simulink model "building_EXAMPLE_v1"  (R2016b)
settings: Solver=ode23tb  StartTime=-building.preruntime+8760*3600  StopTime=building.runtime+8760*3600  MaxStep=600  EnableMultiTasking=on
StartFcn:
  | tic
StopFcn:
  | toc
values from neighbouring files (symbols this model uses):
  building = create_building_automatic(building, modify, import_mode, name_XML, name_EXCEL, name_PHPP, NUMBEROFZONES)    [work_EXAMPLE_v1.m]
undefined symbols (not defined in the file or in its folder): A, B, C, cp, Dd, Dreifach, FluidMix, get_building, ID, MassFlow, p, Pressure, Qdot_C, Qdot_C_energy, Qdot_H, Qdot_H_energy, Qdot_I_electricity, Qdot_I_electricity_energy, Qdot_I_light, Qdot_I_light_energy, Qdot_I_person, Qdot_I_person_energy, Qdot_S, Qdot_S_energy, Qdot_T_ground, Qdot_T_ground_energy, Qdot_T_neighbour, Qdot_T_neighbour_energy, Qdot_T_opaque, Qdot_T_opaque_energy, Qdot_T_window, Qdot_T_window_energy, Qdot_V_infiltration, Qdot_V_infiltration_energy, Qdot_V_mech, Qdot_V_mech_energy, Qdot_V_window, Qdot_V_window_energy, rho, Tc, Temperature, Tr, Ts, Wärmeschutzglas, x_CO2, x_H2O, x_VOC
libraries: carnotUIBK x1931, carnot x83, simulink_extras x22, simulink x12
(part 11 of 35)

== system building_EXAMPLE_v1/HVAC PKOM4/electrical heater 3 ==
  temperature room : Inport
  " " : Constant  Value=0
  "   " : Constant  Value=zeros(1,15)
  Bus Selector5 : BusSelector  OutputSignals=Ts
  Constant 3 : Constant  Value=theta_r_t  VectorParams1D=off
  Constant 9 : Constant  Value=theta_r_t_low  VectorParams1D=off
  Mux1 : Mux  Inputs=[1 1 15 1 1]
  PID_1 : simulink/Continuous/PID Controller  Controller=PI  TimeDomain=Continuous-time  SampleTime=-1  IntegratorMethod=Forward Euler  FilterMethod=Forward Euler  Form=Ideal  UseFilter=on  ControllerParametersSource=internal  P=Kp  I=(1/(Tn*60))  D=0  N=100  InitialConditionSource=internal  InitialConditionForIntegrator=0  InitialConditionForFilter=0  ExternalReset=none  LimitOutput=on  UpperSaturationLimit=1  LowerSaturationLimit=0  LinearizeAsGain=off  AntiWindupMode=clamping  Kb=1  TrackingMode=off  Kt=1  PParamMin=[]  PParamMax=[]  IParamMin=[]  IParamMax=[]  DParamMin=[]  DParamMax=[]  NParamMin=[]  NParamMax=[]  KbParamMin=[]  KbParamMax=[]  KtParamMin=[]  KtParamMax=[]  POutMin=[]  POutMax=[]  IOutMin=[]  IOutMax=[]  DOutMin=[]  DOutMax=[]  NOutMin=[]  NOutMax=[]  KbOutMin=[]  KbOutMax=[]  KtOutMin=[]  KtOutMax=[]  IntegratorOutMin=[]  IntegratorOutMax=[]  FilterOutMin=[]  FilterOutMax=[]  SumOutMin=[]  SumOutMax=[]  SumI1OutMin=[]  SumI1OutMax=[]  SumI2OutMin=[]  SumI2OutMax=[]  SumI3OutMin=[]  SumI3OutMax=[]  SumDOutMin=[]  SumDOutMax=[]  SaturationOutMin=[]  SaturationOutMax=[]  IntegratorContinuousStateAttributes=''  IntegratorStateMustResolveToSignalObject=off  IntegratorRTWStateStorageClass=Auto  FilterContinuousStateAttributes=''  FilterStateMustResolveToSignalObject=off  FilterRTWStateStorageClass=Auto  DifferentiatorICPrevScaledInput=0  DifferentiatorOutMin=[]  DifferentiatorOutMax=[]
  Sum13 : Sum  Inputs=|+-
  Switch : Switch  Criteria=u2 ~= 0
  Transfer Fcn (with initial states) : Subsystem  mask(Transfer Function with Initial States){N=[1], D=[timeconstant_heater  1], X0=0}
      mask prompts: N "Numerator:"; D "Denominator:"; X0 "Initial conditions:"
      mask help: Vector expressions for numerator, and denominator. Coefficients are in descending powers of s.
      mask init:
      | [A,B,C,Dd]=tf2ss(N,D);if (isempty(X0));[m,n]=size(A);X0=zeros(1,m); end;
      mask Help: Specify the initial states for the transfer function.  The state ordering is determined by the m-file tf2ss.  There is no unique mapping of the states in a transfer function to states in a state-space representation.  However, tf2ss will consistently use the same mapping for a given transfer function.
      mask Display: dpoly(N,D,'s')
  Transfer Fcn (with initial states)6 : Subsystem  mask(Transfer Function with Initial States){N=[1], D=[60  1], X0=0}
      mask prompts: N "Numerator:"; D "Denominator:"; X0 "Initial conditions:"
      mask help: Vector expressions for numerator, and denominator. Coefficients are in descending powers of s.
      mask init:
      | [A,B,C,Dd]=tf2ss(N,D);if (isempty(X0));[m,n]=size(A);X0=zeros(1,m); end;
      mask Help: Specify the initial states for the transfer function.  The state ordering is determined by the m-file tf2ss.  There is no unique mapping of the states in a transfer function to states in a state-space representation.  However, tf2ss will consistently use the same mapping for a given transfer function.
      mask Display: dpoly(N,D,'s')
  conv : Gain  Gain=1-part_rad  SaturateOnIntegerOverflow=on  OutDataTypeStr=Inherit: Same as input  ParamDataTypeStr=Inherit: Same as input
  heater : Product
  maximal power : Constant  Value=max_power
  rad : Gain  Gain=part_rad  SaturateOnIntegerOverflow=on  OutDataTypeStr=Inherit: Same as input  ParamDataTypeStr=Inherit: Same as input
  time profile : carnot/Load/General/Repeating_Profile  period=sum(control_time_duration)  rep_seq_t=control_time_values  rep_seq_d=control_time_duration  rep_seq_y=control_time_output
  "[S]" : Outport
  Pel : Outport  Port=2
  wires:
  time profile/1 -> Switch/2
  Switch/1 -> Sum13/1
  Constant 9/1 -> Switch/3
  Constant 3/1 -> Switch/1
  Transfer Fcn (with initial states)/1(Out1) -> Mux1/4, rad/1, conv/1
  Bus Selector5/1 -> Sum13/2  "<Ts>"
  Sum13/1 -> Transfer Fcn (with initial states)6/1(In1)
  heater/1 -> Transfer Fcn (with initial states)/1(In1), Pel/1
  "   "/1 -> Mux1/3
  rad/1 -> Mux1/2
  temperature room/1 -> Bus Selector5/1
  maximal power/1 -> heater/2
  conv/1 -> Mux1/1
  Mux1/1 -> "[S]"/1
  " "/1 -> Mux1/5
  PID_1/1 -> heater/1
  Transfer Fcn (with initial states)6/1(Out1) -> PID_1/1

== system building_EXAMPLE_v1/HVAC PKOM4/electrical heater 4 CONVECTOR ==
  temperature room : Inport
  " " : Constant  Value=0
  "   " : Constant  Value=zeros(1,15)
  Bus Selector5 : BusSelector  OutputSignals=Ts
  Constant 3 : Constant  Value=theta_r_t  VectorParams1D=off
  Constant 9 : Constant  Value=theta_r_t_low  VectorParams1D=off
  Mux1 : Mux  Inputs=[1 1 15 1 1]
  PID_1 : simulink/Continuous/PID Controller  Controller=PI  TimeDomain=Continuous-time  SampleTime=-1  IntegratorMethod=Forward Euler  FilterMethod=Forward Euler  Form=Ideal  UseFilter=on  ControllerParametersSource=internal  P=Kp  I=(1/(Tn*60))  D=0  N=100  InitialConditionSource=internal  InitialConditionForIntegrator=0  InitialConditionForFilter=0  ExternalReset=none  LimitOutput=on  UpperSaturationLimit=1  LowerSaturationLimit=0  LinearizeAsGain=off  AntiWindupMode=clamping  Kb=1  TrackingMode=off  Kt=1  PParamMin=[]  PParamMax=[]  IParamMin=[]  IParamMax=[]  DParamMin=[]  DParamMax=[]  NParamMin=[]  NParamMax=[]  KbParamMin=[]  KbParamMax=[]  KtParamMin=[]  KtParamMax=[]  POutMin=[]  POutMax=[]  IOutMin=[]  IOutMax=[]  DOutMin=[]  DOutMax=[]  NOutMin=[]  NOutMax=[]  KbOutMin=[]  KbOutMax=[]  KtOutMin=[]  KtOutMax=[]  IntegratorOutMin=[]  IntegratorOutMax=[]  FilterOutMin=[]  FilterOutMax=[]  SumOutMin=[]  SumOutMax=[]  SumI1OutMin=[]  SumI1OutMax=[]  SumI2OutMin=[]  SumI2OutMax=[]  SumI3OutMin=[]  SumI3OutMax=[]  SumDOutMin=[]  SumDOutMax=[]  SaturationOutMin=[]  SaturationOutMax=[]  IntegratorContinuousStateAttributes=''  IntegratorStateMustResolveToSignalObject=off  IntegratorRTWStateStorageClass=Auto  FilterContinuousStateAttributes=''  FilterStateMustResolveToSignalObject=off  FilterRTWStateStorageClass=Auto  DifferentiatorICPrevScaledInput=0  DifferentiatorOutMin=[]  DifferentiatorOutMax=[]
  Sum13 : Sum  Inputs=|+-
  Switch : Switch  Criteria=u2 ~= 0
  Transfer Fcn (with initial states) : Subsystem  mask(Transfer Function with Initial States){N=[1], D=[timeconstant_heater  1], X0=0}
      mask prompts: N "Numerator:"; D "Denominator:"; X0 "Initial conditions:"
      mask help: Vector expressions for numerator, and denominator. Coefficients are in descending powers of s.
      mask init:
      | [A,B,C,Dd]=tf2ss(N,D);if (isempty(X0));[m,n]=size(A);X0=zeros(1,m); end;
      mask Help: Specify the initial states for the transfer function.  The state ordering is determined by the m-file tf2ss.  There is no unique mapping of the states in a transfer function to states in a state-space representation.  However, tf2ss will consistently use the same mapping for a given transfer function.
      mask Display: dpoly(N,D,'s')
  Transfer Fcn (with initial states)6 : Subsystem  mask(Transfer Function with Initial States){N=[1], D=[60  1], X0=0}
      mask prompts: N "Numerator:"; D "Denominator:"; X0 "Initial conditions:"
      mask help: Vector expressions for numerator, and denominator. Coefficients are in descending powers of s.
      mask init:
      | [A,B,C,Dd]=tf2ss(N,D);if (isempty(X0));[m,n]=size(A);X0=zeros(1,m); end;
      mask Help: Specify the initial states for the transfer function.  The state ordering is determined by the m-file tf2ss.  There is no unique mapping of the states in a transfer function to states in a state-space representation.  However, tf2ss will consistently use the same mapping for a given transfer function.
      mask Display: dpoly(N,D,'s')
  conv : Gain  Gain=1-part_rad  SaturateOnIntegerOverflow=on  OutDataTypeStr=Inherit: Same as input  ParamDataTypeStr=Inherit: Same as input
  heater : Product
  maximal power : Constant  Value=max_power
  rad : Gain  Gain=part_rad  SaturateOnIntegerOverflow=on  OutDataTypeStr=Inherit: Same as input  ParamDataTypeStr=Inherit: Same as input
  time profile : carnot/Load/General/Repeating_Profile  period=sum(control_time_duration)  rep_seq_t=control_time_values  rep_seq_d=control_time_duration  rep_seq_y=control_time_output
  "[S]" : Outport
  Pel : Outport  Port=2
  wires:
  Transfer Fcn (with initial states)6/1(Out1) -> PID_1/1
  PID_1/1 -> heater/1
  " "/1 -> Mux1/5
  Mux1/1 -> "[S]"/1
  conv/1 -> Mux1/1
  maximal power/1 -> heater/2
  temperature room/1 -> Bus Selector5/1
  rad/1 -> Mux1/2
  "   "/1 -> Mux1/3
  heater/1 -> Pel/1, Transfer Fcn (with initial states)/1(In1)
  Sum13/1 -> Transfer Fcn (with initial states)6/1(In1)
  Bus Selector5/1 -> Sum13/2  "<Ts>"
  Transfer Fcn (with initial states)/1(Out1) -> conv/1, rad/1, Mux1/4
  Constant 3/1 -> Switch/1
  Constant 9/1 -> Switch/3
  Switch/1 -> Sum13/1
  time profile/1 -> Switch/2

== system building_EXAMPLE_v1/HVAC PKOM4/electrical heater 5 ==
  temperature room : Inport
  " " : Constant  Value=0
  "   " : Constant  Value=zeros(1,15)
  Bus Selector5 : BusSelector  OutputSignals=Ts
  Constant 3 : Constant  Value=theta_r_t  VectorParams1D=off
  Constant 9 : Constant  Value=theta_r_t_low  VectorParams1D=off
  Mux1 : Mux  Inputs=[1 1 15 1 1]
  PID_1 : simulink/Continuous/PID Controller  Controller=PI  TimeDomain=Continuous-time  SampleTime=-1  IntegratorMethod=Forward Euler  FilterMethod=Forward Euler  Form=Ideal  UseFilter=on  ControllerParametersSource=internal  P=Kp  I=(1/(Tn*60))  D=0  N=100  InitialConditionSource=internal  InitialConditionForIntegrator=0  InitialConditionForFilter=0  ExternalReset=none  LimitOutput=on  UpperSaturationLimit=1  LowerSaturationLimit=0  LinearizeAsGain=off  AntiWindupMode=clamping  Kb=1  TrackingMode=off  Kt=1  PParamMin=[]  PParamMax=[]  IParamMin=[]  IParamMax=[]  DParamMin=[]  DParamMax=[]  NParamMin=[]  NParamMax=[]  KbParamMin=[]  KbParamMax=[]  KtParamMin=[]  KtParamMax=[]  POutMin=[]  POutMax=[]  IOutMin=[]  IOutMax=[]  DOutMin=[]  DOutMax=[]  NOutMin=[]  NOutMax=[]  KbOutMin=[]  KbOutMax=[]  KtOutMin=[]  KtOutMax=[]  IntegratorOutMin=[]  IntegratorOutMax=[]  FilterOutMin=[]  FilterOutMax=[]  SumOutMin=[]  SumOutMax=[]  SumI1OutMin=[]  SumI1OutMax=[]  SumI2OutMin=[]  SumI2OutMax=[]  SumI3OutMin=[]  SumI3OutMax=[]  SumDOutMin=[]  SumDOutMax=[]  SaturationOutMin=[]  SaturationOutMax=[]  IntegratorContinuousStateAttributes=''  IntegratorStateMustResolveToSignalObject=off  IntegratorRTWStateStorageClass=Auto  FilterContinuousStateAttributes=''  FilterStateMustResolveToSignalObject=off  FilterRTWStateStorageClass=Auto  DifferentiatorICPrevScaledInput=0  DifferentiatorOutMin=[]  DifferentiatorOutMax=[]
  Sum13 : Sum  Inputs=|+-
  Switch : Switch  Criteria=u2 ~= 0
  Transfer Fcn (with initial states) : Subsystem  mask(Transfer Function with Initial States){N=[1], D=[timeconstant_heater  1], X0=0}
      mask prompts: N "Numerator:"; D "Denominator:"; X0 "Initial conditions:"
      mask help: Vector expressions for numerator, and denominator. Coefficients are in descending powers of s.
      mask init:
      | [A,B,C,Dd]=tf2ss(N,D);if (isempty(X0));[m,n]=size(A);X0=zeros(1,m); end;
      mask Help: Specify the initial states for the transfer function.  The state ordering is determined by the m-file tf2ss.  There is no unique mapping of the states in a transfer function to states in a state-space representation.  However, tf2ss will consistently use the same mapping for a given transfer function.
      mask Display: dpoly(N,D,'s')
  Transfer Fcn (with initial states)6 : Subsystem  mask(Transfer Function with Initial States){N=[1], D=[60  1], X0=0}
      mask prompts: N "Numerator:"; D "Denominator:"; X0 "Initial conditions:"
      mask help: Vector expressions for numerator, and denominator. Coefficients are in descending powers of s.
      mask init:
      | [A,B,C,Dd]=tf2ss(N,D);if (isempty(X0));[m,n]=size(A);X0=zeros(1,m); end;
      mask Help: Specify the initial states for the transfer function.  The state ordering is determined by the m-file tf2ss.  There is no unique mapping of the states in a transfer function to states in a state-space representation.  However, tf2ss will consistently use the same mapping for a given transfer function.
      mask Display: dpoly(N,D,'s')
  conv : Gain  Gain=1-part_rad  SaturateOnIntegerOverflow=on  OutDataTypeStr=Inherit: Same as input  ParamDataTypeStr=Inherit: Same as input
  heater : Product
  maximal power : Constant  Value=max_power
  rad : Gain  Gain=part_rad  SaturateOnIntegerOverflow=on  OutDataTypeStr=Inherit: Same as input  ParamDataTypeStr=Inherit: Same as input
  time profile : carnot/Load/General/Repeating_Profile  period=sum(control_time_duration)  rep_seq_t=control_time_values  rep_seq_d=control_time_duration  rep_seq_y=control_time_output
  "[S]" : Outport
  Pel : Outport  Port=2
  wires:
  time profile/1 -> Switch/2
  Switch/1 -> Sum13/1
  Constant 9/1 -> Switch/3
  Constant 3/1 -> Switch/1
  Transfer Fcn (with initial states)/1(Out1) -> Mux1/4, rad/1, conv/1
  Bus Selector5/1 -> Sum13/2  "<Ts>"
  Sum13/1 -> Transfer Fcn (with initial states)6/1(In1)
  heater/1 -> Transfer Fcn (with initial states)/1(In1), Pel/1
  "   "/1 -> Mux1/3
  rad/1 -> Mux1/2
  temperature room/1 -> Bus Selector5/1
  maximal power/1 -> heater/2
  conv/1 -> Mux1/1
  Mux1/1 -> "[S]"/1
  " "/1 -> Mux1/5
  PID_1/1 -> heater/1
  Transfer Fcn (with initial states)6/1(Out1) -> PID_1/1

== system building_EXAMPLE_v1/HVAC PKOM4/electrical heater 6 ==
  temperature room : Inport
  " " : Constant  Value=0
  "   " : Constant  Value=zeros(1,15)
  Bus Selector5 : BusSelector  OutputSignals=Ts
  Constant 3 : Constant  Value=theta_r_t  VectorParams1D=off
  Constant 9 : Constant  Value=theta_r_t_low  VectorParams1D=off
  Mux1 : Mux  Inputs=[1 1 15 1 1]
  PID_1 : simulink/Continuous/PID Controller  Controller=PI  TimeDomain=Continuous-time  SampleTime=-1  IntegratorMethod=Forward Euler  FilterMethod=Forward Euler  Form=Ideal  UseFilter=on  ControllerParametersSource=internal  P=Kp  I=(1/(Tn*60))  D=0  N=100  InitialConditionSource=internal  InitialConditionForIntegrator=0  InitialConditionForFilter=0  ExternalReset=none  LimitOutput=on  UpperSaturationLimit=1  LowerSaturationLimit=0  LinearizeAsGain=off  AntiWindupMode=clamping  Kb=1  TrackingMode=off  Kt=1  PParamMin=[]  PParamMax=[]  IParamMin=[]  IParamMax=[]  DParamMin=[]  DParamMax=[]  NParamMin=[]  NParamMax=[]  KbParamMin=[]  KbParamMax=[]  KtParamMin=[]  KtParamMax=[]  POutMin=[]  POutMax=[]  IOutMin=[]  IOutMax=[]  DOutMin=[]  DOutMax=[]  NOutMin=[]  NOutMax=[]  KbOutMin=[]  KbOutMax=[]  KtOutMin=[]  KtOutMax=[]  IntegratorOutMin=[]  IntegratorOutMax=[]  FilterOutMin=[]  FilterOutMax=[]  SumOutMin=[]  SumOutMax=[]  SumI1OutMin=[]  SumI1OutMax=[]  SumI2OutMin=[]  SumI2OutMax=[]  SumI3OutMin=[]  SumI3OutMax=[]  SumDOutMin=[]  SumDOutMax=[]  SaturationOutMin=[]  SaturationOutMax=[]  IntegratorContinuousStateAttributes=''  IntegratorStateMustResolveToSignalObject=off  IntegratorRTWStateStorageClass=Auto  FilterContinuousStateAttributes=''  FilterStateMustResolveToSignalObject=off  FilterRTWStateStorageClass=Auto  DifferentiatorICPrevScaledInput=0  DifferentiatorOutMin=[]  DifferentiatorOutMax=[]
  Sum13 : Sum  Inputs=|+-
  Switch : Switch  Criteria=u2 ~= 0
  Transfer Fcn (with initial states) : Subsystem  mask(Transfer Function with Initial States){N=[1], D=[timeconstant_heater  1], X0=0}
      mask prompts: N "Numerator:"; D "Denominator:"; X0 "Initial conditions:"
      mask help: Vector expressions for numerator, and denominator. Coefficients are in descending powers of s.
      mask init:
      | [A,B,C,Dd]=tf2ss(N,D);if (isempty(X0));[m,n]=size(A);X0=zeros(1,m); end;
      mask Help: Specify the initial states for the transfer function.  The state ordering is determined by the m-file tf2ss.  There is no unique mapping of the states in a transfer function to states in a state-space representation.  However, tf2ss will consistently use the same mapping for a given transfer function.
      mask Display: dpoly(N,D,'s')
  Transfer Fcn (with initial states)6 : Subsystem  mask(Transfer Function with Initial States){N=[1], D=[60  1], X0=0}
      mask prompts: N "Numerator:"; D "Denominator:"; X0 "Initial conditions:"
      mask help: Vector expressions for numerator, and denominator. Coefficients are in descending powers of s.
      mask init:
      | [A,B,C,Dd]=tf2ss(N,D);if (isempty(X0));[m,n]=size(A);X0=zeros(1,m); end;
      mask Help: Specify the initial states for the transfer function.  The state ordering is determined by the m-file tf2ss.  There is no unique mapping of the states in a transfer function to states in a state-space representation.  However, tf2ss will consistently use the same mapping for a given transfer function.
      mask Display: dpoly(N,D,'s')
  conv : Gain  Gain=1-part_rad  SaturateOnIntegerOverflow=on  OutDataTypeStr=Inherit: Same as input  ParamDataTypeStr=Inherit: Same as input
  heater : Product
  maximal power : Constant  Value=max_power
  rad : Gain  Gain=part_rad  SaturateOnIntegerOverflow=on  OutDataTypeStr=Inherit: Same as input  ParamDataTypeStr=Inherit: Same as input
  time profile : carnot/Load/General/Repeating_Profile  period=sum(control_time_duration)  rep_seq_t=control_time_values  rep_seq_d=control_time_duration  rep_seq_y=control_time_output
  "[S]" : Outport
  Pel : Outport  Port=2
  wires:
  Transfer Fcn (with initial states)6/1(Out1) -> PID_1/1
  PID_1/1 -> heater/1
  " "/1 -> Mux1/5
  Mux1/1 -> "[S]"/1
  conv/1 -> Mux1/1
  maximal power/1 -> heater/2
  temperature room/1 -> Bus Selector5/1
  rad/1 -> Mux1/2
  "   "/1 -> Mux1/3
  heater/1 -> Pel/1, Transfer Fcn (with initial states)/1(In1)
  Sum13/1 -> Transfer Fcn (with initial states)6/1(In1)
  Bus Selector5/1 -> Sum13/2  "<Ts>"
  Transfer Fcn (with initial states)/1(Out1) -> conv/1, rad/1, Mux1/4
  Constant 3/1 -> Switch/1
  Constant 9/1 -> Switch/3
  Switch/1 -> Sum13/1
  time profile/1 -> Switch/2

== system building_EXAMPLE_v1/HVAC PKOM4/electrical heater 7 ==
  temperature room : Inport
  " " : Constant  Value=0
  "   " : Constant  Value=zeros(1,15)
  Bus Selector5 : BusSelector  OutputSignals=Ts
  Constant 3 : Constant  Value=theta_r_t  VectorParams1D=off
  Constant 9 : Constant  Value=theta_r_t_low  VectorParams1D=off
  Mux1 : Mux  Inputs=[1 1 15 1 1]
  PID_1 : simulink/Continuous/PID Controller  Controller=PI  TimeDomain=Continuous-time  SampleTime=-1  IntegratorMethod=Forward Euler  FilterMethod=Forward Euler  Form=Ideal  UseFilter=on  ControllerParametersSource=internal  P=Kp  I=(1/(Tn*60))  D=0  N=100  InitialConditionSource=internal  InitialConditionForIntegrator=0  InitialConditionForFilter=0  ExternalReset=none  LimitOutput=on  UpperSaturationLimit=1  LowerSaturationLimit=0  LinearizeAsGain=off  AntiWindupMode=clamping  Kb=1  TrackingMode=off  Kt=1  PParamMin=[]  PParamMax=[]  IParamMin=[]  IParamMax=[]  DParamMin=[]  DParamMax=[]  NParamMin=[]  NParamMax=[]  KbParamMin=[]  KbParamMax=[]  KtParamMin=[]  KtParamMax=[]  POutMin=[]  POutMax=[]  IOutMin=[]  IOutMax=[]  DOutMin=[]  DOutMax=[]  NOutMin=[]  NOutMax=[]  KbOutMin=[]  KbOutMax=[]  KtOutMin=[]  KtOutMax=[]  IntegratorOutMin=[]  IntegratorOutMax=[]  FilterOutMin=[]  FilterOutMax=[]  SumOutMin=[]  SumOutMax=[]  SumI1OutMin=[]  SumI1OutMax=[]  SumI2OutMin=[]  SumI2OutMax=[]  SumI3OutMin=[]  SumI3OutMax=[]  SumDOutMin=[]  SumDOutMax=[]  SaturationOutMin=[]  SaturationOutMax=[]  IntegratorContinuousStateAttributes=''  IntegratorStateMustResolveToSignalObject=off  IntegratorRTWStateStorageClass=Auto  FilterContinuousStateAttributes=''  FilterStateMustResolveToSignalObject=off  FilterRTWStateStorageClass=Auto  DifferentiatorICPrevScaledInput=0  DifferentiatorOutMin=[]  DifferentiatorOutMax=[]
  Sum13 : Sum  Inputs=|+-
  Switch : Switch  Criteria=u2 ~= 0
  Transfer Fcn (with initial states) : Subsystem  mask(Transfer Function with Initial States){N=[1], D=[timeconstant_heater  1], X0=0}
      mask prompts: N "Numerator:"; D "Denominator:"; X0 "Initial conditions:"
      mask help: Vector expressions for numerator, and denominator. Coefficients are in descending powers of s.
      mask init:
      | [A,B,C,Dd]=tf2ss(N,D);if (isempty(X0));[m,n]=size(A);X0=zeros(1,m); end;
      mask Help: Specify the initial states for the transfer function.  The state ordering is determined by the m-file tf2ss.  There is no unique mapping of the states in a transfer function to states in a state-space representation.  However, tf2ss will consistently use the same mapping for a given transfer function.
      mask Display: dpoly(N,D,'s')
  Transfer Fcn (with initial states)6 : Subsystem  mask(Transfer Function with Initial States){N=[1], D=[60  1], X0=0}
      mask prompts: N "Numerator:"; D "Denominator:"; X0 "Initial conditions:"
      mask help: Vector expressions for numerator, and denominator. Coefficients are in descending powers of s.
      mask init:
      | [A,B,C,Dd]=tf2ss(N,D);if (isempty(X0));[m,n]=size(A);X0=zeros(1,m); end;
      mask Help: Specify the initial states for the transfer function.  The state ordering is determined by the m-file tf2ss.  There is no unique mapping of the states in a transfer function to states in a state-space representation.  However, tf2ss will consistently use the same mapping for a given transfer function.
      mask Display: dpoly(N,D,'s')
  conv : Gain  Gain=1-part_rad  SaturateOnIntegerOverflow=on  OutDataTypeStr=Inherit: Same as input  ParamDataTypeStr=Inherit: Same as input
  heater : Product
  maximal power : Constant  Value=max_power
  rad : Gain  Gain=part_rad  SaturateOnIntegerOverflow=on  OutDataTypeStr=Inherit: Same as input  ParamDataTypeStr=Inherit: Same as input
  time profile : carnot/Load/General/Repeating_Profile  period=sum(control_time_duration)  rep_seq_t=control_time_values  rep_seq_d=control_time_duration  rep_seq_y=control_time_output
  "[S]" : Outport
  Pel : Outport  Port=2
  wires:
  time profile/1 -> Switch/2
  Switch/1 -> Sum13/1
  Constant 9/1 -> Switch/3
  Constant 3/1 -> Switch/1
  Transfer Fcn (with initial states)/1(Out1) -> Mux1/4, rad/1, conv/1
  Bus Selector5/1 -> Sum13/2  "<Ts>"
  Sum13/1 -> Transfer Fcn (with initial states)6/1(In1)
  heater/1 -> Transfer Fcn (with initial states)/1(In1), Pel/1
  "   "/1 -> Mux1/3
  rad/1 -> Mux1/2
  temperature room/1 -> Bus Selector5/1
  maximal power/1 -> heater/2
  conv/1 -> Mux1/1
  Mux1/1 -> "[S]"/1
  " "/1 -> Mux1/5
  PID_1/1 -> heater/1
  Transfer Fcn (with initial states)6/1(Out1) -> PID_1/1

== system building_EXAMPLE_v1/HVAC PKOM4/heatpump heating ==
  controller state : Inport
  setpoint frequency : Inport  Port=2
  h_exh : Inport  Port=3
  controller postheater : Inport  Port=4
  Add3 : Sum  Inputs=+-
  Add4 : Sum
  Add5 : Sum
  Constant1 : Constant  Value=0
  Constant2 : Constant
  Gain1 : Gain  Gain=.5
  Gain2 : Gain  Gain=.5
  Ground{1..6} (6 alike) : Ground
  Mux2 : Mux  Inputs=2
  Mux5 : Mux  Inputs=[1 2 1 2 5 1 5 1 1]
  PT1 _ 1 : simulink_extras/Additional Linear/Transfer Fcn (with initial outputs)  N=[1]  D=[heatpump.timeconstant(1) 1]  Y0=0  U0=0
  PT1 _ 2 : simulink_extras/Additional Linear/Transfer Fcn (with initial outputs)  N=[1]  D=[heatpump.timeconstant(2) 1]  Y0=0  U0=0
  PT1 _ 3 : simulink_extras/Additional Linear/Transfer Fcn (with initial outputs)  N=[1]  D=[60 1]  Y0=0  U0=0
  PT1 _ 4 : simulink_extras/Additional Linear/Transfer Fcn (with initial outputs)  N=[1]  D=[hvac.postheater.timeconstant 1]  Y0=0  U0=0
  PT1 _ 7 : simulink_extras/Additional Linear/Transfer Fcn (with initial outputs)  N=[1]  D=[heatpump.timeconstant(1) 1]  Y0=0  U0=0
  PT1 _ 8 : simulink_extras/Additional Linear/Transfer Fcn (with initial outputs)  N=[1]  D=[heatpump.timeconstant(2) 1]  Y0=0  U0=0
  calc_Pel_compressor : Subsystem  mask{pol=heatpump.Pel_compressor}
  calc_Pel_compressor_useable : Subsystem  mask{pol=heatpump.Pel_compressor_useable}
  calc_Qdot_sup : Subsystem  mask{pol=heatpump.Qdot_sup}
  calc_deicing : Subsystem  mask{pol=heatpump.deicing}
  heating mode : RelationalOperator  Operator===  OutDataTypeStr=boolean  RndMeth=Simplest
  limit power1 : Saturate  UpperLimit=1e4  LowerLimit=0
  limit power2 : Saturate  UpperLimit=1e4  LowerLimit=0
  limit power3 : Saturate  UpperLimit=1e4  LowerLimit=0
  on/off BU : Switch  Threshold=1
  on/off HP : Switch  Threshold=1
  power postheater : Gain  Gain=hvac.postheater.power
  stop : Gain  Gain=0
  "[S]_losses_HP" : Outport
  deicing : Outport  Port=2
  Qdot_sup : Outport  Port=3
  Qdot_sup_postheater : Outport  Port=4
  Pel_compressor : Outport  Port=5
  Pel_compressor_useable : Outport  Port=6
  Pel_postheater : Outport  Port=7
  wires:
  on/off HP/1 -> calc_Pel_compressor/1(u), calc_deicing/1(u), calc_Pel_compressor_useable/1(u), calc_Qdot_sup/1(u)
  calc_Pel_compressor_useable/1(y) -> limit power3/1  "Pel_compressor_useable"
  calc_Pel_compressor/1(y) -> limit power2/1  "Pel_compressor"
  Ground6/1 -> Mux5/7
  Gain2/1 -> Qdot_sup/1, Mux5/8  "Qdot_sup"
  Mux5/1 -> "[S]_losses_HP"/1
  Ground3/1 -> Mux5/4
  calc_Qdot_sup/1(y) -> limit power1/1  "Qdot_sup"
  PT1 _ 1/1 -> Add5/1
  PT1 _ 2/1 -> Add5/2
  PT1 _ 8/1 -> Add4/2
  Add3/1 -> PT1 _ 2/1, PT1 _ 1/1  "Qdot_losses"
  Ground4/1 -> Mux5/3
  Gain1/1 -> Mux5/1, Mux5/6
  Ground2/1 -> Mux5/2
  PT1 _ 7/1 -> Add4/1
  Ground1/1 -> Mux5/5
  Add4/1 -> Gain2/1
  Add5/1 -> Gain1/1
  stop/1 -> on/off HP/3
  controller state/1 -> heating mode/1
  heating mode/1 -> on/off BU/2, on/off HP/2
  Constant2/1 -> heating mode/2
  setpoint frequency/1 -> Mux2/2
  h_exh/1 -> Mux2/1
  Mux2/1 -> stop/1, on/off HP/1
  Ground5/1 -> Mux5/9
  calc_deicing/1(deicing time) -> PT1 _ 3/1
  PT1 _ 3/1 -> deicing/1
  limit power3/1 -> Pel_compressor_useable/1, Add3/2
  limit power1/1 -> PT1 _ 8/1, PT1 _ 7/1  "Qdot_sup"
  limit power2/1 -> Pel_compressor/1, Add3/1
  on/off BU/1 -> power postheater/1
  power postheater/1 -> PT1 _ 4/1, Pel_postheater/1
  PT1 _ 4/1 -> Qdot_sup_postheater/1
  controller postheater/1 -> on/off BU/1
  Constant1/1 -> on/off BU/3

== system building_EXAMPLE_v1/HVAC electrical heaters/Subsystem ==
  setpoint : Inport
  AIB : Inport  Port=2
  Bus Selector5 : BusSelector  OutputSignals=Tc,p,x_H2O
  Fcn : Fcn  Expr=(u(1)-30)/20*0.5
  Sum : Sum  Inputs=|+-
  Transfer Fcn (with initial states)6 : carnotUIBK/HVAC/electrical heater/Transfer Fcn (with initial states)6  N=[1]  D=[7200 1]  X0=0
  reduce temperature : Saturate  LowerLimit=-0.25
  x2RelHum_UIBK : carnot/Basic/Material_Properties/x2RelHum
  setpoint corr : Outport
  wires:
  Transfer Fcn (with initial states)6/1 -> Sum/2
  Bus Selector5/2 -> x2RelHum_UIBK/2  "<p>"
  AIB/1 -> Bus Selector5/1
  Bus Selector5/1 -> x2RelHum_UIBK/1  "<Tc>"
  Bus Selector5/3 -> x2RelHum_UIBK/3  "<x_H2O>"
  Sum/1 -> setpoint corr/1
  setpoint/1 -> Sum/1
  reduce temperature/1 -> Transfer Fcn (with initial states)6/1
  Fcn/1 -> reduce temperature/1
  x2RelHum_UIBK/1 -> Fcn/1

== system building_EXAMPLE_v1/HVAC electrical heaters/Subsystem1 ==
  setpoint : Inport
  AIB : Inport  Port=2
  Bus Selector5 : BusSelector  OutputSignals=Tc,p,x_H2O
  Fcn : Fcn  Expr=(u(1)-30)/20*0.5
  Sum : Sum  Inputs=|+-
  Transfer Fcn (with initial states)6 : carnotUIBK/HVAC/electrical heater/Transfer Fcn (with initial states)6  N=[1]  D=[7200 1]  X0=0
  reduce temperature : Saturate  LowerLimit=-0.25
  x2RelHum_UIBK : carnot/Basic/Material_Properties/x2RelHum
  setpoint corr : Outport
  wires:
  x2RelHum_UIBK/1 -> Fcn/1
  Fcn/1 -> reduce temperature/1
  reduce temperature/1 -> Transfer Fcn (with initial states)6/1
  setpoint/1 -> Sum/1
  Sum/1 -> setpoint corr/1
  Bus Selector5/3 -> x2RelHum_UIBK/3  "<x_H2O>"
  Bus Selector5/1 -> x2RelHum_UIBK/1  "<Tc>"
  AIB/1 -> Bus Selector5/1
  Bus Selector5/2 -> x2RelHum_UIBK/2  "<p>"
  Transfer Fcn (with initial states)6/1 -> Sum/2

== system building_EXAMPLE_v1/HVAC electrical heaters/Subsystem2 ==
  setpoint : Inport
  AIB : Inport  Port=2
  Bus Selector5 : BusSelector  OutputSignals=Tc,p,x_H2O
  Fcn : Fcn  Expr=(u(1)-30)/20*0.5
  Sum : Sum  Inputs=|+-
  Transfer Fcn (with initial states)6 : carnotUIBK/HVAC/electrical heater/Transfer Fcn (with initial states)6  N=[1]  D=[7200 1]  X0=0
  reduce temperature : Saturate  LowerLimit=-0.25
  x2RelHum_UIBK : carnot/Basic/Material_Properties/x2RelHum
  setpoint corr : Outport
  wires:
  Transfer Fcn (with initial states)6/1 -> Sum/2
  Bus Selector5/2 -> x2RelHum_UIBK/2  "<p>"
  AIB/1 -> Bus Selector5/1
  Bus Selector5/1 -> x2RelHum_UIBK/1  "<Tc>"
  Bus Selector5/3 -> x2RelHum_UIBK/3  "<x_H2O>"
  Sum/1 -> setpoint corr/1
  setpoint/1 -> Sum/1
  reduce temperature/1 -> Transfer Fcn (with initial states)6/1
  Fcn/1 -> reduce temperature/1
  x2RelHum_UIBK/1 -> Fcn/1

== system building_EXAMPLE_v1/HVAC electrical heaters/Subsystem3 ==
  setpoint : Inport
  AIB : Inport  Port=2
  Bus Selector5 : BusSelector  OutputSignals=Tc,p,x_H2O
  Fcn : Fcn  Expr=(u(1)-30)/20*0.5
  Sum : Sum  Inputs=|+-
  Transfer Fcn (with initial states)6 : carnotUIBK/HVAC/electrical heater/Transfer Fcn (with initial states)6  N=[1]  D=[7200 1]  X0=0
  reduce temperature : Saturate  LowerLimit=-0.25
  x2RelHum_UIBK : carnot/Basic/Material_Properties/x2RelHum
  setpoint corr : Outport
  wires:
  x2RelHum_UIBK/1 -> Fcn/1
  Fcn/1 -> reduce temperature/1
  reduce temperature/1 -> Transfer Fcn (with initial states)6/1
  setpoint/1 -> Sum/1
  Sum/1 -> setpoint corr/1
  Bus Selector5/3 -> x2RelHum_UIBK/3  "<x_H2O>"
  Bus Selector5/1 -> x2RelHum_UIBK/1  "<Tc>"
  AIB/1 -> Bus Selector5/1
  Bus Selector5/2 -> x2RelHum_UIBK/2  "<p>"
  Transfer Fcn (with initial states)6/1 -> Sum/2

== system building_EXAMPLE_v1/HVAC electrical heaters/Subsystem4 ==
  setpoint : Inport
  AIB : Inport  Port=2
  Bus Selector5 : BusSelector  OutputSignals=Tc,p,x_H2O
  Fcn : Fcn  Expr=(u(1)-30)/20*0.5
  Sum : Sum  Inputs=|+-
  Transfer Fcn (with initial states)6 : carnotUIBK/HVAC/electrical heater/Transfer Fcn (with initial states)6  N=[1]  D=[7200 1]  X0=0
  reduce temperature : Saturate  LowerLimit=-0.25
  x2RelHum_UIBK : carnot/Basic/Material_Properties/x2RelHum
  setpoint corr : Outport
  wires:
  Transfer Fcn (with initial states)6/1 -> Sum/2
  Bus Selector5/2 -> x2RelHum_UIBK/2  "<p>"
  AIB/1 -> Bus Selector5/1
  Bus Selector5/1 -> x2RelHum_UIBK/1  "<Tc>"
  Bus Selector5/3 -> x2RelHum_UIBK/3  "<x_H2O>"
  Sum/1 -> setpoint corr/1
  setpoint/1 -> Sum/1
  reduce temperature/1 -> Transfer Fcn (with initial states)6/1
  Fcn/1 -> reduce temperature/1
  x2RelHum_UIBK/1 -> Fcn/1

== system building_EXAMPLE_v1/HVAC electrical heaters/Subsystem5 ==
  setpoint : Inport
  AIB : Inport  Port=2
  Bus Selector5 : BusSelector  OutputSignals=Tc,p,x_H2O
  Fcn : Fcn  Expr=(u(1)-30)/20*0.5
  Sum : Sum  Inputs=|+-
  Transfer Fcn (with initial states)6 : carnotUIBK/HVAC/electrical heater/Transfer Fcn (with initial states)6  N=[1]  D=[7200 1]  X0=0
  reduce temperature : Saturate  LowerLimit=-0.25
  x2RelHum_UIBK : carnot/Basic/Material_Properties/x2RelHum
  setpoint corr : Outport
  wires:
  x2RelHum_UIBK/1 -> Fcn/1
  Fcn/1 -> reduce temperature/1
  reduce temperature/1 -> Transfer Fcn (with initial states)6/1
  setpoint/1 -> Sum/1
  Sum/1 -> setpoint corr/1
  Bus Selector5/3 -> x2RelHum_UIBK/3  "<x_H2O>"
  Bus Selector5/1 -> x2RelHum_UIBK/1  "<Tc>"
  AIB/1 -> Bus Selector5/1
  Bus Selector5/2 -> x2RelHum_UIBK/2  "<p>"
  Transfer Fcn (with initial states)6/1 -> Sum/2

== system building_EXAMPLE_v1/HVAC electrical heaters/Subsystem6 ==
  setpoint : Inport
  AIB : Inport  Port=2
  Bus Selector5 : BusSelector  OutputSignals=Tc,p,x_H2O
  Fcn : Fcn  Expr=(u(1)-30)/20*0.5
  Sum : Sum  Inputs=|+-
  Transfer Fcn (with initial states)6 : carnotUIBK/HVAC/electrical heater/Transfer Fcn (with initial states)6  N=[1]  D=[7200 1]  X0=0
  reduce temperature : Saturate  LowerLimit=-0.25
  x2RelHum_UIBK : carnot/Basic/Material_Properties/x2RelHum
  setpoint corr : Outport
  wires:
  Transfer Fcn (with initial states)6/1 -> Sum/2
  Bus Selector5/2 -> x2RelHum_UIBK/2  "<p>"
  AIB/1 -> Bus Selector5/1
  Bus Selector5/1 -> x2RelHum_UIBK/1  "<Tc>"
  Bus Selector5/3 -> x2RelHum_UIBK/3  "<x_H2O>"
  Sum/1 -> setpoint corr/1
  setpoint/1 -> Sum/1
  reduce temperature/1 -> Transfer Fcn (with initial states)6/1
  Fcn/1 -> reduce temperature/1
  x2RelHum_UIBK/1 -> Fcn/1

== system building_EXAMPLE_v1/HVAC pipes/Pipes_inlet ==
  AIBkueche : Inport
  AIBGang : Inport  Port=2
  THBvent1 : Inport  Port=3
  Add : Sum  Inputs=+++++
  Bus Selector3 : BusSelector  OutputSignals=Ts
  Bus Selector5 : BusSelector  OutputSignals=Ts
  THB_split3 : Subsystem
  THB_split4 : Subsystem  AncestorBlock=carnot/misc/THV_template
  pipe_gang_com_kind_wohnz : carnotUIBK/HVAC/pipe  pipe=hvac.pipe_in_gang_com_kind_wohnz
  pipe_gang_common : carnotUIBK/HVAC/pipe  pipe=hvac.pipe_in_gang_common
  pipe_gang_eltern : carnotUIBK/HVAC/pipe  pipe=hvac.pipe_in_gang_eltern
  pipe_gang_kind : carnotUIBK/HVAC/pipe  pipe=hvac.pipe_in_gang_kind
  pipe_gang_wohnz : carnotUIBK/HVAC/pipe  pipe=hvac.pipe_in_gang_wohnz
  pipe_kueche : carnotUIBK/HVAC/pipe  pipe=hvac.pipe_in_kueche
  S Gang : Outport
  THB eltern : Outport  Port=2
  THB kind : Outport  Port=3
  THB wohnz : Outport  Port=4
  S Kueche : Outport  Port=5
  wires:
  AIBkueche/1 -> Bus Selector5/1
  AIBGang/1 -> Bus Selector3/1
  THBvent1/1 -> pipe_kueche/2
  pipe_kueche/1 -> pipe_gang_common/2
  Bus Selector5/1 -> pipe_kueche/1  "<Ts>"
  Bus Selector3/1 -> pipe_gang_kind/1, pipe_gang_wohnz/1, pipe_gang_com_kind_wohnz/1, pipe_gang_eltern/1, pipe_gang_common/1  "<Ts>"
  pipe_kueche/2 -> S Kueche/1
  THB_split3/1(THB1out) -> pipe_gang_com_kind_wohnz/2
  THB_split3/2(THB2out) -> pipe_gang_eltern/2
  pipe_gang_common/1 -> THB_split3/1(THBin)
  pipe_gang_kind/1 -> THB kind/1
  pipe_gang_wohnz/1 -> THB wohnz/1
  pipe_gang_eltern/1 -> THB eltern/1
  pipe_gang_com_kind_wohnz/1 -> THB_split4/1(THBin)
  THB_split4/1(THB1out) -> pipe_gang_kind/2
  THB_split4/2(THB2out) -> pipe_gang_wohnz/2
  Add/1 -> S Gang/1
  pipe_gang_kind/2 -> Add/1
  pipe_gang_wohnz/2 -> Add/2
  pipe_gang_com_kind_wohnz/2 -> Add/3
  pipe_gang_eltern/2 -> Add/4
  pipe_gang_common/2 -> Add/5

== system building_EXAMPLE_v1/HVAC pipes/Pipes_outlet ==
  AIBkueche : Inport
  AIBGang : Inport  Port=2
  AIBbad : Inport  Port=3
  Add : Sum
  Bus Selector1 : BusSelector  OutputSignals=Tc,rho,p,x_H2O
  Bus Selector2 : BusSelector  OutputSignals=Tc,rho,p,x_H2O
  Bus Selector3 : BusSelector  OutputSignals=Ts
  Subsystem : Subsystem
  mix : Subsystem
  pipe_gang_bad : carnotUIBK/HVAC/pipe  pipe=hvac.pipe_out_gang_bad
  pipe_gang_common : carnotUIBK/HVAC/pipe  pipe=hvac.pipe_out_gang_common
  pipe_gang_kueche : carnotUIBK/HVAC/pipe  pipe=hvac.pipe_out_gang_kueche
  pipe_kueche_common : carnotUIBK/HVAC/pipe  pipe=hvac.pipe_out_kueche_common
  THB_extract : Outport
  S Bad : Outport  Port=2
  S Kueche : Outport  Port=3
  S Gang : Outport  Port=4
  wires:
  AIBkueche/1 -> Bus Selector1/1
  Bus Selector1/1 -> pipe_gang_kueche/1, Subsystem/5(T_kueche)  "<Tc>"
  AIBbad/1 -> Bus Selector2/1
  Bus Selector2/2 -> Subsystem/2(rho_bad)  "<rho>"
  Bus Selector2/3 -> Subsystem/3(P_bad)  "<p>"
  Bus Selector1/2 -> Subsystem/6(rho_kueche)  "<rho>"
  Bus Selector1/3 -> Subsystem/7(P_kueche)  "<p>"
  AIBGang/1 -> Bus Selector3/1
  Bus Selector1/4 -> Subsystem/8(x_H2O_kueche)  "<x_H2O>"
  Bus Selector2/4 -> Subsystem/4(x_H2O_bad)  "<x_H2O>"
  Bus Selector2/1 -> Subsystem/1(T_bad), pipe_gang_bad/1  "<Tc>"
  pipe_gang_common/1 -> pipe_kueche_common/2
  pipe_kueche_common/1 -> THB_extract/1
  Bus Selector3/1 -> pipe_gang_common/1, pipe_kueche_common/1  "<Ts>"
  pipe_gang_bad/2 -> S Bad/1
  pipe_gang_kueche/2 -> S Kueche/1
  Subsystem/1(THB_bad) -> pipe_gang_bad/2
  pipe_gang_bad/1 -> mix/1(THB_1)
  pipe_gang_kueche/1 -> mix/2(THB_2)
  Subsystem/2(THB_kuche) -> pipe_gang_kueche/2
  mix/1(THB_common) -> pipe_gang_common/2
  Add/1 -> S Gang/1
  pipe_kueche_common/2 -> Add/1
  pipe_gang_common/2 -> Add/2

== system building_EXAMPLE_v1/HVAC pipes/ventilation_inlet1_z1 ==
  "[AIB]" : Inport
  THBin : Inport  Port=2
  MASSin : Inport  Port=3
  Bus Selector : BusSelector  OutputSignals=Temperature,MassFlow
  Bus Selector1 : BusSelector  OutputSignals=Tc
  Gain : Gain  Gain=perc_Vdot_tot
  Ground1 : Ground
  Ground2 : Ground
  Ground6 : Ground
  Mux1 : Mux  Inputs=[1 2 1 2 5 1 7]
  Product4 : Product  Inputs=3  SaturateOnIntegerOverflow=on  InputSameDT=on  OutDataTypeStr=Inherit: Same as first input
  Sum : Sum  Inputs=-+  SaturateOnIntegerOverflow=on  InputSameDT=on  OutDataTypeStr=Inherit: Same as first input
  cp : Constant  Value=1006.8
  "[S]" : Outport
  wires:
  THBin/1 -> Bus Selector/1
  Sum/1 -> Product4/2  "dT"
  Mux1/1 -> "[S]"/1
  "[AIB]"/1 -> Bus Selector1/1
  Bus Selector1/1 -> Sum/1  "<Tc>"
  MASSin/1 -> Gain/1
  Ground6/1 -> Mux1/7
  Ground2/1 -> Mux1/2
  Ground1/1 -> Mux1/5
  Product4/1 -> Mux1/1, Mux1/6
  cp/1 -> Product4/1
  Bus Selector/1 -> Sum/2  "<Temperature>"
  Bus Selector/2 -> Mux1/3, Product4/3  "<MassFlow>"
  Gain/1 -> Mux1/4

== system building_EXAMPLE_v1/HVAC pipes/ventilation_inlet1_z10 ==
  "[AIB]" : Inport
  THBin : Inport  Port=2
  MASSin : Inport  Port=3
  Bus Selector : BusSelector  OutputSignals=Temperature,MassFlow
  Bus Selector1 : BusSelector  OutputSignals=Tc
  Gain : Gain  Gain=perc_Vdot_tot
  Ground1 : Ground
  Ground2 : Ground
  Ground6 : Ground
  Mux1 : Mux  Inputs=[1 2 1 2 5 1 7]
  Product4 : Product  Inputs=3  SaturateOnIntegerOverflow=on  InputSameDT=on  OutDataTypeStr=Inherit: Same as first input
  Sum : Sum  Inputs=-+  SaturateOnIntegerOverflow=on  InputSameDT=on  OutDataTypeStr=Inherit: Same as first input
  cp : Constant  Value=1006.8
  "[S]" : Outport
  wires:
  THBin/1 -> Bus Selector/1
  Sum/1 -> Product4/2  "dT"
  Mux1/1 -> "[S]"/1
  "[AIB]"/1 -> Bus Selector1/1
  Bus Selector1/1 -> Sum/1  "<Tc>"
  MASSin/1 -> Gain/1
  Ground6/1 -> Mux1/7
  Ground2/1 -> Mux1/2
  Ground1/1 -> Mux1/5
  Product4/1 -> Mux1/1, Mux1/6
  cp/1 -> Product4/1
  Bus Selector/1 -> Sum/2  "<Temperature>"
  Bus Selector/2 -> Mux1/3, Product4/3  "<MassFlow>"
  Gain/1 -> Mux1/4

== system building_EXAMPLE_v1/HVAC pipes/ventilation_inlet1_z2 ==
  "[AIB]" : Inport
  THBin : Inport  Port=2
  MASSin : Inport  Port=3
  Bus Selector : BusSelector  OutputSignals=Temperature,MassFlow
  Bus Selector1 : BusSelector  OutputSignals=Tc
  Gain : Gain  Gain=perc_Vdot_tot
  Ground1 : Ground
  Ground2 : Ground
  Ground6 : Ground
  Mux1 : Mux  Inputs=[1 2 1 2 5 1 7]
  Product4 : Product  Inputs=3  SaturateOnIntegerOverflow=on  InputSameDT=on  OutDataTypeStr=Inherit: Same as first input
  Sum : Sum  Inputs=-+  SaturateOnIntegerOverflow=on  InputSameDT=on  OutDataTypeStr=Inherit: Same as first input
  cp : Constant  Value=1006.8
  "[S]" : Outport
  wires:
  THBin/1 -> Bus Selector/1
  Sum/1 -> Product4/2  "dT"
  Mux1/1 -> "[S]"/1
  "[AIB]"/1 -> Bus Selector1/1
  Bus Selector1/1 -> Sum/1  "<Tc>"
  MASSin/1 -> Gain/1
  Ground6/1 -> Mux1/7
  Ground2/1 -> Mux1/2
  Ground1/1 -> Mux1/5
  Product4/1 -> Mux1/1, Mux1/6
  cp/1 -> Product4/1
  Bus Selector/1 -> Sum/2  "<Temperature>"
  Bus Selector/2 -> Mux1/3, Product4/3  "<MassFlow>"
  Gain/1 -> Mux1/4

== system building_EXAMPLE_v1/HVAC pipes/ventilation_inlet1_z3 ==
  "[AIB]" : Inport
  THBin : Inport  Port=2
  MASSin : Inport  Port=3
  Bus Selector : BusSelector  OutputSignals=Temperature,MassFlow
  Bus Selector1 : BusSelector  OutputSignals=Tc
  Gain : Gain  Gain=perc_Vdot_tot
  Ground1 : Ground
  Ground2 : Ground
  Ground6 : Ground
  Mux1 : Mux  Inputs=[1 2 1 2 5 1 7]
  Product4 : Product  Inputs=3  SaturateOnIntegerOverflow=on  InputSameDT=on  OutDataTypeStr=Inherit: Same as first input
  Sum : Sum  Inputs=-+  SaturateOnIntegerOverflow=on  InputSameDT=on  OutDataTypeStr=Inherit: Same as first input
  cp : Constant  Value=1006.8
  "[S]" : Outport
  wires:
  THBin/1 -> Bus Selector/1
  Sum/1 -> Product4/2  "dT"
  Mux1/1 -> "[S]"/1
  "[AIB]"/1 -> Bus Selector1/1
  Bus Selector1/1 -> Sum/1  "<Tc>"
  MASSin/1 -> Gain/1
  Ground6/1 -> Mux1/7
  Ground2/1 -> Mux1/2
  Ground1/1 -> Mux1/5
  Product4/1 -> Mux1/1, Mux1/6
  cp/1 -> Product4/1
  Bus Selector/1 -> Sum/2  "<Temperature>"
  Bus Selector/2 -> Mux1/3, Product4/3  "<MassFlow>"
  Gain/1 -> Mux1/4

== system building_EXAMPLE_v1/HVAC pipes/ventilation_inlet1_z4 ==
  "[AIB]" : Inport
  THBin : Inport  Port=2
  MASSin : Inport  Port=3
  Bus Selector : BusSelector  OutputSignals=Temperature,MassFlow
  Bus Selector1 : BusSelector  OutputSignals=Tc
  Gain : Gain  Gain=perc_Vdot_tot
  Ground1 : Ground
  Ground2 : Ground
  Ground6 : Ground
  Mux1 : Mux  Inputs=[1 2 1 2 5 1 7]
  Product4 : Product  Inputs=3  SaturateOnIntegerOverflow=on  InputSameDT=on  OutDataTypeStr=Inherit: Same as first input
  Sum : Sum  Inputs=-+  SaturateOnIntegerOverflow=on  InputSameDT=on  OutDataTypeStr=Inherit: Same as first input
  cp : Constant  Value=1006.8
  "[S]" : Outport
  wires:
  THBin/1 -> Bus Selector/1
  Sum/1 -> Product4/2  "dT"
  Mux1/1 -> "[S]"/1
  "[AIB]"/1 -> Bus Selector1/1
  Bus Selector1/1 -> Sum/1  "<Tc>"
  MASSin/1 -> Gain/1
  Ground6/1 -> Mux1/7
  Ground2/1 -> Mux1/2
  Ground1/1 -> Mux1/5
  Product4/1 -> Mux1/1, Mux1/6
  cp/1 -> Product4/1
  Bus Selector/1 -> Sum/2  "<Temperature>"
  Bus Selector/2 -> Mux1/3, Product4/3  "<MassFlow>"
  Gain/1 -> Mux1/4

== system building_EXAMPLE_v1/HVAC pipes/ventilation_inlet1_z5 ==
  "[AIB]" : Inport
  THBin : Inport  Port=2
  MASSin : Inport  Port=3
  Bus Selector : BusSelector  OutputSignals=Temperature,MassFlow
  Bus Selector1 : BusSelector  OutputSignals=Tc
  Gain : Gain  Gain=perc_Vdot_tot
  Ground1 : Ground
  Ground2 : Ground
  Ground6 : Ground
  Mux1 : Mux  Inputs=[1 2 1 2 5 1 7]
  Product4 : Product  Inputs=3  SaturateOnIntegerOverflow=on  InputSameDT=on  OutDataTypeStr=Inherit: Same as first input
  Sum : Sum  Inputs=-+  SaturateOnIntegerOverflow=on  InputSameDT=on  OutDataTypeStr=Inherit: Same as first input
  cp : Constant  Value=1006.8
  "[S]" : Outport
  wires:
  THBin/1 -> Bus Selector/1
  Sum/1 -> Product4/2  "dT"
  Mux1/1 -> "[S]"/1
  "[AIB]"/1 -> Bus Selector1/1
  Bus Selector1/1 -> Sum/1  "<Tc>"
  MASSin/1 -> Gain/1
  Ground6/1 -> Mux1/7
  Ground2/1 -> Mux1/2
  Ground1/1 -> Mux1/5
  Product4/1 -> Mux1/1, Mux1/6
  cp/1 -> Product4/1
  Bus Selector/1 -> Sum/2  "<Temperature>"
  Bus Selector/2 -> Mux1/3, Product4/3  "<MassFlow>"
  Gain/1 -> Mux1/4

== system building_EXAMPLE_v1/HVAC pipes/ventilation_inlet1_z6 ==
  "[AIB]" : Inport
  THBin : Inport  Port=2
  MASSin : Inport  Port=3
  Bus Selector : BusSelector  OutputSignals=Temperature,MassFlow
  Bus Selector1 : BusSelector  OutputSignals=Tc
  Gain : Gain  Gain=perc_Vdot_tot
  Ground1 : Ground
  Ground2 : Ground
  Ground6 : Ground
  Mux1 : Mux  Inputs=[1 2 1 2 5 1 7]
  Product4 : Product  Inputs=3  SaturateOnIntegerOverflow=on  InputSameDT=on  OutDataTypeStr=Inherit: Same as first input
  Sum : Sum  Inputs=-+  SaturateOnIntegerOverflow=on  InputSameDT=on  OutDataTypeStr=Inherit: Same as first input
  cp : Constant  Value=1006.8
  "[S]" : Outport
  wires:
  THBin/1 -> Bus Selector/1
  Sum/1 -> Product4/2  "dT"
  Mux1/1 -> "[S]"/1
  "[AIB]"/1 -> Bus Selector1/1
  Bus Selector1/1 -> Sum/1  "<Tc>"
  MASSin/1 -> Gain/1
  Ground6/1 -> Mux1/7
  Ground2/1 -> Mux1/2
  Ground1/1 -> Mux1/5
  Product4/1 -> Mux1/1, Mux1/6
  cp/1 -> Product4/1
  Bus Selector/1 -> Sum/2  "<Temperature>"
  Bus Selector/2 -> Mux1/3, Product4/3  "<MassFlow>"
  Gain/1 -> Mux1/4

== system building_EXAMPLE_v1/HVAC pipes/ventilation_inlet1_z7 ==
  "[AIB]" : Inport
  THBin : Inport  Port=2
  MASSin : Inport  Port=3
  Bus Selector : BusSelector  OutputSignals=Temperature,MassFlow
  Bus Selector1 : BusSelector  OutputSignals=Tc
  Gain : Gain  Gain=perc_Vdot_tot
  Ground1 : Ground
  Ground2 : Ground
  Ground6 : Ground
  Mux1 : Mux  Inputs=[1 2 1 2 5 1 7]
  Product4 : Product  Inputs=3  SaturateOnIntegerOverflow=on  InputSameDT=on  OutDataTypeStr=Inherit: Same as first input
  Sum : Sum  Inputs=-+  SaturateOnIntegerOverflow=on  InputSameDT=on  OutDataTypeStr=Inherit: Same as first input
  cp : Constant  Value=1006.8
  "[S]" : Outport
  wires:
  THBin/1 -> Bus Selector/1
  Sum/1 -> Product4/2  "dT"
  Mux1/1 -> "[S]"/1
  "[AIB]"/1 -> Bus Selector1/1
  Bus Selector1/1 -> Sum/1  "<Tc>"
  MASSin/1 -> Gain/1
  Ground6/1 -> Mux1/7
  Ground2/1 -> Mux1/2
  Ground1/1 -> Mux1/5
  Product4/1 -> Mux1/1, Mux1/6
  cp/1 -> Product4/1
  Bus Selector/1 -> Sum/2  "<Temperature>"
  Bus Selector/2 -> Mux1/3, Product4/3  "<MassFlow>"
  Gain/1 -> Mux1/4

== system building_EXAMPLE_v1/HVAC pipes/ventilation_inlet1_z8 ==
  "[AIB]" : Inport
  THBin : Inport  Port=2
  MASSin : Inport  Port=3
  Bus Selector : BusSelector  OutputSignals=Temperature,MassFlow
  Bus Selector1 : BusSelector  OutputSignals=Tc
  Gain : Gain  Gain=perc_Vdot_tot
  Ground1 : Ground
  Ground2 : Ground
  Ground6 : Ground
  Mux1 : Mux  Inputs=[1 2 1 2 5 1 7]
  Product4 : Product  Inputs=3  SaturateOnIntegerOverflow=on  InputSameDT=on  OutDataTypeStr=Inherit: Same as first input
  Sum : Sum  Inputs=-+  SaturateOnIntegerOverflow=on  InputSameDT=on  OutDataTypeStr=Inherit: Same as first input
  cp : Constant  Value=1006.8
  "[S]" : Outport
  wires:
  THBin/1 -> Bus Selector/1
  Sum/1 -> Product4/2  "dT"
  Mux1/1 -> "[S]"/1
  "[AIB]"/1 -> Bus Selector1/1
  Bus Selector1/1 -> Sum/1  "<Tc>"
  MASSin/1 -> Gain/1
  Ground6/1 -> Mux1/7
  Ground2/1 -> Mux1/2
  Ground1/1 -> Mux1/5
  Product4/1 -> Mux1/1, Mux1/6
  cp/1 -> Product4/1
  Bus Selector/1 -> Sum/2  "<Temperature>"
  Bus Selector/2 -> Mux1/3, Product4/3  "<MassFlow>"
  Gain/1 -> Mux1/4

== system building_EXAMPLE_v1/HVAC pipes/ventilation_inlet1_z9 ==
  "[AIB]" : Inport
  THBin : Inport  Port=2
  MASSin : Inport  Port=3
  Bus Selector : BusSelector  OutputSignals=Temperature,MassFlow
  Bus Selector1 : BusSelector  OutputSignals=Tc
  Gain : Gain  Gain=perc_Vdot_tot
  Ground1 : Ground
  Ground2 : Ground
  Ground6 : Ground
  Mux1 : Mux  Inputs=[1 2 1 2 5 1 7]
  Product4 : Product  Inputs=3  SaturateOnIntegerOverflow=on  InputSameDT=on  OutDataTypeStr=Inherit: Same as first input
  Sum : Sum  Inputs=-+  SaturateOnIntegerOverflow=on  InputSameDT=on  OutDataTypeStr=Inherit: Same as first input
  cp : Constant  Value=1006.8
  "[S]" : Outport
  wires:
  THBin/1 -> Bus Selector/1
  Sum/1 -> Product4/2  "dT"
  Mux1/1 -> "[S]"/1
  "[AIB]"/1 -> Bus Selector1/1
  Bus Selector1/1 -> Sum/1  "<Tc>"
  MASSin/1 -> Gain/1
  Ground6/1 -> Mux1/7
  Ground2/1 -> Mux1/2
  Ground1/1 -> Mux1/5
  Product4/1 -> Mux1/1, Mux1/6
  cp/1 -> Product4/1
  Bus Selector/1 -> Sum/2  "<Temperature>"
  Bus Selector/2 -> Mux1/3, Product4/3  "<MassFlow>"
  Gain/1 -> Mux1/4

== system building_EXAMPLE_v1/HVAC pipes/ventilation_outlet1_z1 ==
  note: no energy flux
  note: see energy balance
  "[AIB]" : Inport
  Vdot : Inport  Port=2
  (kg/m³).(m³/h) : Product
  Bus Selector1 : BusSelector  OutputSignals=rho,Tc,p
  Bus Selector2 : BusSelector  OutputSignals=x_H2O
  Bus Selector3 : BusSelector  OutputSignals=x_CO2
  Fcn1 : Fcn  Expr=u / (1+u)
  Fcn2 : Fcn  Expr=u / (1+u)
  Gain : Gain  Gain=perc_Vdot_tot
  Gain1 : Gain  Gain=-1
  Gain3 : Gain  Gain=-1
  Gain4 : Gain  Gain=-1
  Ground{1..5} (5 alike) : Ground
  Mux1 : Mux  Inputs=[1 2 1 1 1 5 1 7]
  create_THB : Subsystem  mask(create THV){fluid=2, dia=0.125, hgt=0, mID=1}
      mask prompts: dia "diameter [m]"; hgt "Geodetic height in m"; mID "Calculation mode"
      mask help:
      | Create a THB with the variable input T and mdot. The other value can be set as constants in the mask.
      | Calculation mode:
      |     1 ..  9999 no pressure drop (dp)
      | 10001 .. 19999 dp caused by flowrate
      | 20001 .. inf   dp by flowrate and static height
      mask init:
      | dia = max(dia, 0.001);
      mask Help: web(fullfile(path_carnot('help'),'basic_create_THB.html'),'-helpbrowser')
  h/s : Gain  Gain=1/3600
  kg/s : Product
  kg/s1 : Product
  "[S]" : Outport
  THBout : Outport  Port=2  InitialOutput=0
  wires:
  Mux1/1 -> "[S]"/1
  Gain/1 -> (kg/m³).(m³/h)/2
  (kg/m³).(m³/h)/1 -> h/s/1
  h/s/1 -> create_THB/1(mdot), kg/s1/1, kg/s/1, Gain4/1
  Bus Selector2/1 -> create_THB/4(mix), Fcn2/1  "<x_H2O>"
  kg/s/1 -> Gain3/1
  Gain3/1 -> Mux1/4
  Ground4/1 -> Mux1/1
  Ground5/1 -> Mux1/6
  Gain4/1 -> Mux1/3
  Fcn2/1 -> kg/s/2
  Fcn1/1 -> kg/s1/2
  kg/s1/1 -> Gain1/1
  Gain1/1 -> Mux1/5
  "[AIB]"/1 -> Bus Selector1/1, Bus Selector3/1, Bus Selector2/1
  Bus Selector1/1 -> (kg/m³).(m³/h)/1  "<rho>"
  Bus Selector3/1 -> Fcn1/1  "<x_CO2>"
  Ground1/1 -> Mux1/7
  Ground2/1 -> Mux1/8
  Ground3/1 -> Mux1/2
  Vdot/1 -> Gain/1
  Bus Selector1/2 -> create_THB/2(T)  "<Tc>"
  Bus Selector1/3 -> create_THB/3(p)  "<p>"
  create_THB/1(THB) -> THBout/1
